simulink model "SM_3_x_Vm_Gsm"  (R2021b)
settings: Solver=VariableStepAuto  StartTime=0.0  StopTime=5  RelTol=1e-3
settings Model: Creator=sama1402  LastModifiedBy=levm1106

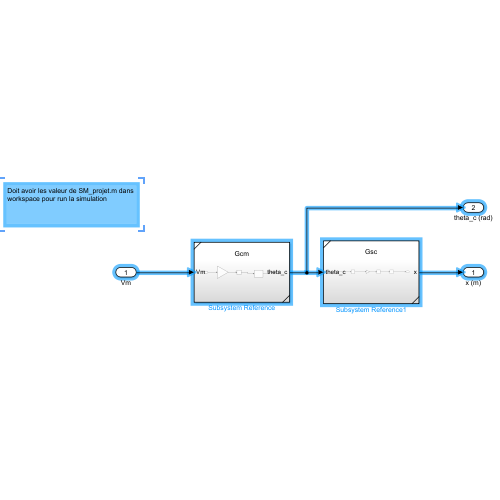
[thumbnail: Simulink's stored preview of the top-level diagram]
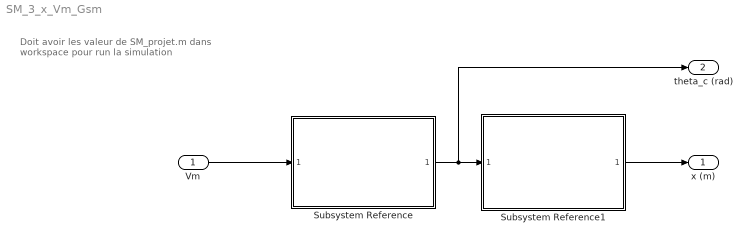
== system SM_3_x_Vm_Gsm ==
  note: Doit avoir les valeur de SM_projet.m dans workspace pour run la simulation
  Vm : Inport
  Subsystem Reference : Subsystem  ReferencedSubsystem=Gcm
  Subsystem Reference1 : Subsystem  ReferencedSubsystem=Gsc
  x (m) : Outport
  theta_c (rad) : Outport  Port=2
  wires:
  Subsystem Reference/1 -> theta_c (rad)/1, Subsystem Reference1/1
  Vm/1 -> Subsystem Reference/1
  Subsystem Reference1/1 -> x (m)/1
